simulink model "nlmpc_ZonePcm_3x"  (R2020b)
settings: Solver=VariableStepAuto  StartTime=0.0  StopTime=86400*2  RelTol=1e-6
values from neighbouring files (symbols this model uses):
  Ts = 900    [NLMPC_ZonePcm_3x.m]
libraries: mpclib x1
settings Model: Creator=taoy  LastModifiedBy=taoy
settings SolverCC: AlgebraicLoopSolver=LineSearch

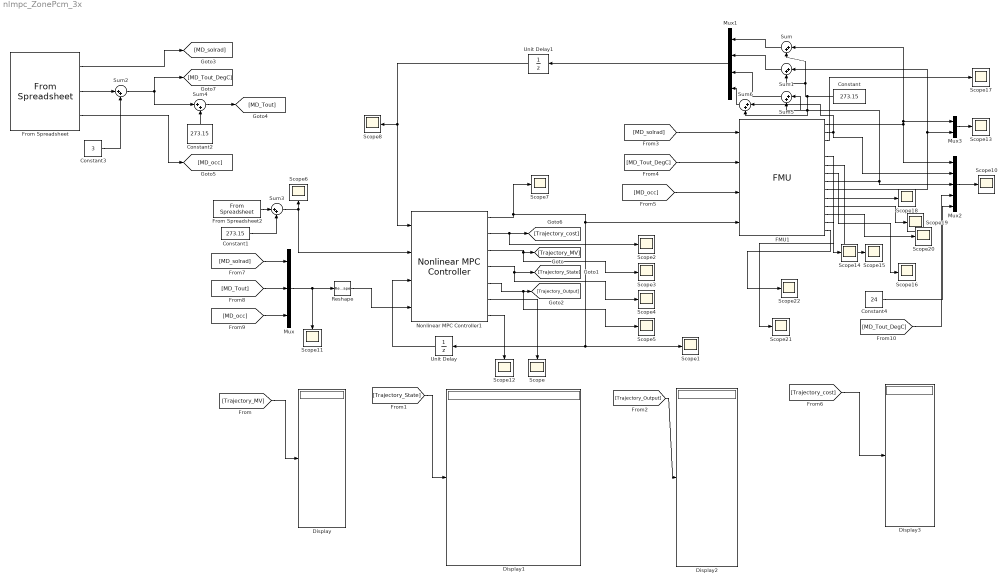
== system nlmpc_ZonePcm_3x ==
  Constant : Constant  Value=273.15
  Constant1 : Constant  Value=273.15
  Constant2 : Constant  Value=273.15
  Constant3 : Constant  Value=3
  Constant4 : Constant  Value=24
  Display{,1..3} (4 alike) : Display
  FMU1 : FMU  FMUName=PCM_zone_update_new_2.fmu  FMUMode=CoSimulation  system=struct('p_ambient',101325,'T_ambient',293.15,'g',9.80665,'m_flow_start',0,'eps_m_flow',0.0001,'dp_small',1,'m_flow_small',0.01)  TairInit=20  mPC_demo4_1=struct('TAirInit_2',20,'CO2Init',400,'RExt',2.0,'RInt',0.05,'tmass',25,'imass',17.89,'shgc',1.985,'CO2n',400,'CO2pp',0.039,'maxVent',1746,'vent',1746,'occ_gain',20.0,'maxHeat',1310,'prescribedHeatFlow',struct('T_ref',293.15,'alpha',0),'occHeatGain',struct('T_ref',293.15,'alpha',0),'Vi',121.625,'occheff',1.0,'Vinf',50,'airMix_new',struct('h_to_s',struct('k',0.0002777777777777778),'AirRhoCp',struct('k',1206.0),'multiProduct',struct('significantDigits',int32(8)),'prescribedHeatFlow',struct('T_ref',293.15,'alpha',0),'add1',struct('k1',1,'k2',-1)),'integrator',struct('k',1,'y_start',0),'Tve',21)  aHU_PCM_one_stack_NoData=struct('PCM1',struct('Tinit',22.0,'heatCapacitor',struct('cp_s',2000,'cp_l',2000,'hf_pcm',140000,'m_pcm',1),'convection_coefficient1',struct('m_PCM_2',100,'k_a',0.02364,'rho_a',1.288,'my_a',1.729E-05,'Pr_a',0.7344,'L_CSM',0.45,'H_c',0.0015,'Nu_rest',7.54),'thermalConductor',struct('G_2',15),'Area',struct('k',0.135),'Lf',struct('Bh',2.118,'Bc',18.37,'Tmc',294.71,'Tmh',295.46999999999997,'vh',2.804,'vc',31.11)),'rho',struct('k',1.288),'boundary',struct('X',[0.01,0.99],'m_flow',0,'T',293.15),'gain1',struct('k',0.0002777777777777778),'gain2',struct('k',0.010416666666666666),'bou',struct('X',[0.01,0.99],'p',101325,'h',45300.945),'vol',struct('p_start',101325,'T_start',293.15,'X_start',[0.01,0.99],'m_flow_nominal',0.0036,'V',0.00010125000000000001))  add=struct('k1',-1,'k2',1)  cp=struct('k',0.00036908333333333335)  multiProduct=struct('significantDigits',int32(3))  const=struct('k',0)  const1=struct('k',0)  const2=struct('k',24)  gain=struct('k',96)  gain1=struct('k',3600)  zeroOrderHold=struct('samplePeriod',60,'startTime',0)  zeroOrderHold1=struct('samplePeriod',60,'startTime',0)  zeroOrderHold2=struct('samplePeriod',60,'startTime',0)  mask(PCM_zone_update_new_2 [Co-Simulation, v2.0]){}
      mask Display:
      | disp('PCM_zone_update_new_2');
      | port_label('output',1,'Tin');
      | port_label('output',2,'Tsup');
      | port_label('output',3,'H');
      | port_label('output',4,'dHdT');
      | port_label('output',5,'Qc');
      | port_label('output',6,'qc');
      | port_label('output',7,'Qsup');
      | port_label('output',8,'Tpcm');
      | port_label('output',9,'Tinterior');
      | port_label('output',10,'y1');
      | port_label('output',11,'y2');
      | port_label('output',12,'y3');
      | port_label('output',13,'Vair_out');
      | port_label('output',14,'k');
      | port_label('input',1,'solrad');
      | port_label('input',2,'Tout');
      | port_label('input',3,'occ');
      | port_label('input',4,'Vair');
  From Spreadsheet : FromSpreadsheet  FileName=meas_q.csv  SheetName=meas_q  SampleTime=-1
  From Spreadsheet2 : FromSpreadsheet  FileName=C:\Users\taoy\Desktop\NLMPC_pcm_toKF - new-data-ssm\data\Tset_7days.csv  SheetName=Tset_7days  SampleTime=900
  Mux : Mux  Inputs=3
  Mux1 : Mux
  Mux2 : Mux  Inputs=5
  Mux3 : Mux  Inputs=2
  Nonlinear MPC Controller1 : mpclib/Nonlinear MPC Controller  SCDEnableBlockLinearizationSpecification=on  nlmpcobj=nlobj_new_3x  UseObjectTs=on  UseMEX=off  md_enabled=on  mvtarget_enabled=off  param_enabled=off  cost_enabled=on  mvseq_enabled=on  stateseq_enabled=on  ovseq_enabled=on  slack_enabled=on  status_enabled=on  ov_min=off  ov_max=off  mv_min=off  mv_max=off  mvrate_min=off  mvrate_max=off  state_min=off  state_max=off  ov_weight=off  mv_weight=off  mvrate_weight=off  ecr_weight=off  nlp_initialize=off
  Reshape : Reshape  OutputDimensionality=Row vector (2-D)
  Scope{,1..8,10..22} (22 alike) : Scope
  Sum{,1..6} (7 alike) : Sum  Inputs=|++
  Unit Delay : UnitDelay  SampleTime=Ts  HasFrameUpgradeWarning=on
  Unit Delay1 : UnitDelay  InitialCondition=[293.15 293.15 288.15 288.15]  SampleTime=Ts  HasFrameUpgradeWarning=on
  wires:
  Nonlinear MPC Controller1/3 -> Scope3/1, [Trajectory_MV]
  Nonlinear MPC Controller1/4 -> Scope4/1, [Trajectory_State]
  Nonlinear MPC Controller1/5 -> Scope5/1, [Trajectory_Output]
  [Trajectory_MV] -> Display/1
  [Trajectory_State] -> Display1/1
  [Trajectory_Output] -> Display2/1
  From Spreadsheet/1 -> [MD_solrad]
  [Trajectory_cost] -> Display3/1
  [MD_solrad] -> Mux/1
  Mux/1 -> Reshape/1, Scope11/1
  Reshape/1 -> Nonlinear MPC Controller1/4
  Unit Delay/1 -> Nonlinear MPC Controller1/3
  Mux1/1 -> Unit Delay1/1
  [MD_solrad] -> FMU1/1
  Nonlinear MPC Controller1/2 -> Scope2/1, [Trajectory_cost]
  Constant/1 -> Sum5/2, Sum6/2, Sum/2, Sum1/2
  FMU1/1 -> Mux2/1, Mux3/1, Sum/1
  FMU1/9 -> Mux3/2, Sum1/1
  Sum/1 -> Mux1/1
  Sum1/1 -> Mux1/2
  [MD_Tout] -> Mux/2
  Mux2/1 -> Scope10/1
  Unit Delay1/1 -> Nonlinear MPC Controller1/1, Scope8/1
  Constant2/1 -> Sum4/2
  Sum4/1 -> [MD_Tout]
  From Spreadsheet2/1 -> Sum3/1
  Constant1/1 -> Sum3/2
  Sum3/1 -> Nonlinear MPC Controller1/2, Scope6/1
  Nonlinear MPC Controller1/6 -> Scope/1
  Nonlinear MPC Controller1/7 -> Scope12/1
  Mux3/1 -> Scope13/1
  FMU1/2 -> Mux2/2, Sum6/1
  [MD_Tout_DegC] -> Mux2/4
  FMU1/5 -> Scope14/1
  FMU1/6 -> Scope15/1
  FMU1/7 -> Scope16/1
  FMU1/3 -> Scope17/1
  From Spreadsheet/2 -> Sum2/1
  Sum2/1 -> Sum4/1, [MD_Tout_DegC]
  Constant3/1 -> Sum2/2
  [MD_Tout_DegC] -> FMU1/2
  FMU1/8 -> Mux2/3, Sum5/1
  Sum5/1 -> Mux1/3
  Nonlinear MPC Controller1/1 -> FMU1/4, Scope1/1, Unit Delay/1, Scope7/1
  FMU1/10 -> Scope18/1
  FMU1/11 -> Scope19/1
  FMU1/12 -> Scope20/1
  Constant4/1 -> Mux2/5
  Sum6/1 -> Mux1/4
  [MD_occ] -> FMU1/3
  [MD_occ] -> Mux/3
  From Spreadsheet/3 -> [MD_occ]
  FMU1/13 -> Scope21/1
  FMU1/14 -> Scope22/1
